simulink model "VehicleModel"  (R2022a)
settings: Solver=VariableStepAuto  StartTime=0.0  StopTime=30  RelTol=1e-3
libraries: simulink x2
settings Model: Creator=raghe  LastModifiedBy=raghe

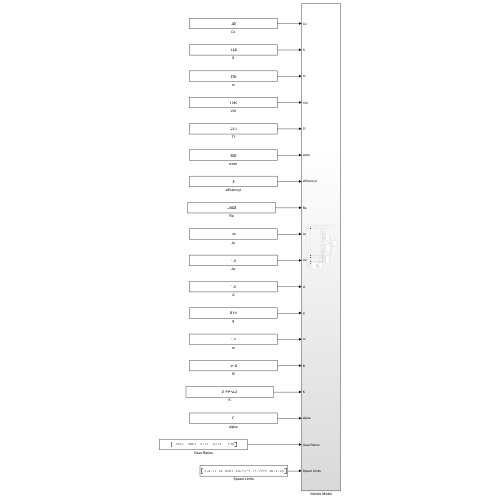
[thumbnail: Simulink's stored preview of the top-level diagram]
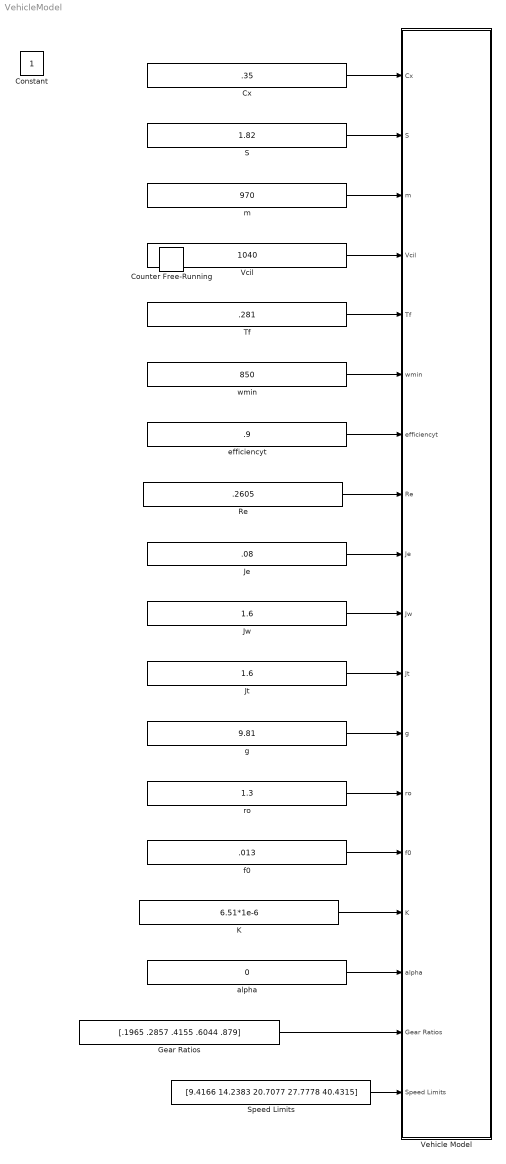
== system VehicleModel ==
  Cx : Constant  Value=.35
  Gear Ratios : Constant  Value=[.1965 .2857 .4155 .6044 .879]
  Je : Constant  Value=.08
  Jt : Constant  Value=1.6
  Jw : Constant  Value=1.6
  K : Constant  Value=6.51*1e-6
  Re : Constant  Value=.2605
  S : Constant  Value=1.82
  Speed Limits : Constant  Value=[9.4166 14.2383 20.7077 27.7778 40.4315]
  Tf : Constant  Value=.281
  Vcil : Constant  Value=1040
  Vehicle Model : Subsystem
  alpha : Constant  Value=0
  efficiencyt : Constant  Value=.9
  f0 : Constant  Value=.013
  g : Constant  Value=9.81
  m : Constant  Value=970
  ro : Constant  Value=1.3
  wmin : Constant  Value=850
  Constant : Constant  IOType=siggen
  Counter Free-Running : simulink/Sources/Counter Free-Running  IOType=siggen  NumBits=16  tsamp=-1
  wires:
  f0/1 -> Vehicle Model/14(f0)
  Vcil/1 -> Vehicle Model/4(Vcil)
  S/1 -> Vehicle Model/2(S)
  g/1 -> Vehicle Model/12(g)
  Re/1 -> Vehicle Model/8(Re)
  Jw/1 -> Vehicle Model/10(Jw)
  efficiencyt/1 -> Vehicle Model/7(efficiencyt)
  Speed Limits/1 -> Vehicle Model/18(Speed Limits)
  Gear Ratios/1 -> Vehicle Model/17(Gear Ratios)
  Je/1 -> Vehicle Model/9(Je)
  Jt/1 -> Vehicle Model/11(Jt)
  Cx/1 -> Vehicle Model/1(Cx)
  ro/1 -> Vehicle Model/13(ro)
  m/1 -> Vehicle Model/3(m)
  K/1 -> Vehicle Model/15(K)
  Tf/1 -> Vehicle Model/5(Tf)
  wmin/1 -> Vehicle Model/6(wmin)
  alpha/1 -> Vehicle Model/16(alpha)

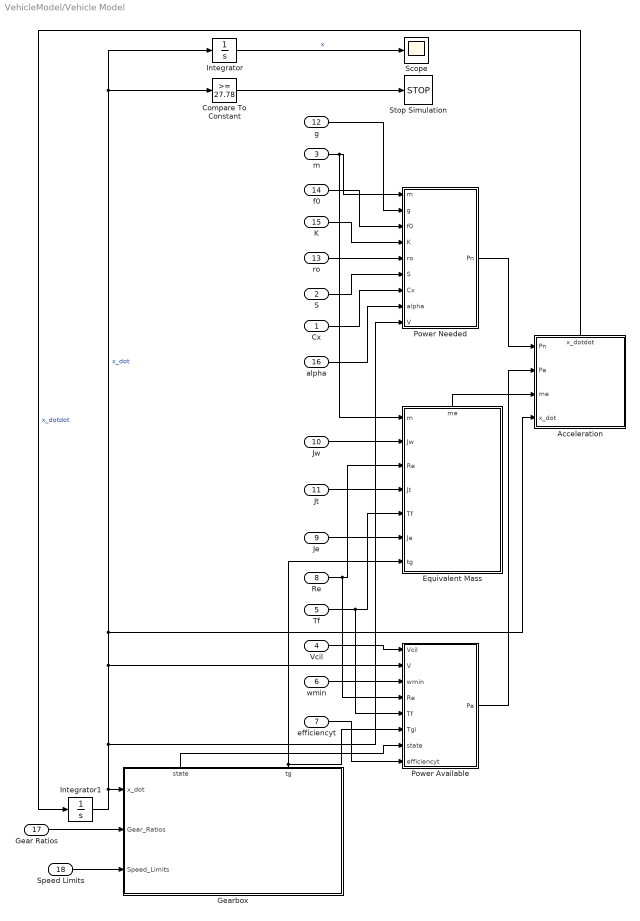
== system VehicleModel/Vehicle Model ==
  Cx : Inport
  S : Inport  Port=2
  m : Inport  Port=3
  Vcil : Inport  Port=4
  Tf : Inport  Port=5
  wmin : Inport  Port=6
  efficiencyt : Inport  Port=7
  Re : Inport  Port=8
  Je : Inport  Port=9
  Jw : Inport  Port=10
  Jt : Inport  Port=11
  g : Inport  Port=12
  ro : Inport  Port=13
  f0 : Inport  Port=14
  K : Inport  Port=15
  alpha : Inport  Port=16
  Gear Ratios : Inport  Port=17
  Speed Limits : Inport  Port=18
  Acceleration : Subsystem
      settings: PortSchema="{\"entries\":[{\"content\":{\"sides\":[{\"content\":{\"connectorIds\":[\"In1\",\"In2\",\"In3\",\"In4\"]},\"type\":\"ConnectorPlacement.EquallySpacedRectSide\",\"uuid\":\"0dac4d62-4e6e-48b9-89ab-502b66d42413\"},{\"content\":{\"connectorIds\":[],\"side\":\"RIGHT\"},\"type\":\"ConnectorPlacement.EquallySpacedRectSide\",\"uuid\":\"bb08bafa-9960-47e7-83c1-b5fcb0a564c6\"},{\"content\":{\"connectorIds\":[\"Out1\"],\"side\":\"TOP\"},\"type\":\"ConnectorPlacement.EquallySpacedRectSide\",\"uuid\":\"4c185d07-b6f8-491a-a2fd-e996dab8f11e\"}]},\"type\":\"ConnectorPlacement.EquallySpacedConnector\",\"uuid\":\"e46381f1-f24e-482b-af6c-f43e86b41e95\"}],\"packageUris\":[\"http://schema.mathworks.com/mf0/Connector/R2020b\"],\"version\":\"1.0\"}"
  Compare To Constant : simulink/Logic and Bit Operations/Compare To Constant  relop=>=  const=27.78  OutDataTypeStr=boolean
  Equivalent Mass : Subsystem
      settings: PortSchema="{\"entries\":[{\"content\":{\"sides\":[{\"content\":{\"connectorIds\":[\"In1\",\"In2\",\"In3\",\"In4\",\"In5\",\"In6\",\"In7\"]},\"type\":\"ConnectorPlacement.EquallySpacedRectSide\",\"uuid\":\"afdafb77-b6a4-4e1f-90ff-c5f4f1bf2fe0\"},{\"content\":{\"connectorIds\":[],\"side\":\"RIGHT\"},\"type\":\"ConnectorPlacement.EquallySpacedRectSide\",\"uuid\":\"5fc42340-ce7c-45bd-a822-e10069a1a8a1\"},{\"content\":{\"connectorIds\":[\"Out1\"],\"side\":\"TOP\"},\"type\":\"ConnectorPlacement.EquallySpacedRectSide\",\"uuid\":\"3dabd7ae-5836-444f-ba7f-aa28a5c4c2aa\"}]},\"type\":\"ConnectorPlacement.EquallySpacedConnector\",\"uuid\":\"25790886-3118-4358-89e2-ebbe2ff8cd9d\"}],\"packageUris\":[\"http://schema.mathworks.com/mf0/Connector/R2020b\"],\"version\":\"1.0\"}"
  Gearbox : Stateflow chart  TreatAsAtomicUnit=on
      settings: PortSchema="{\"entries\":[{\"content\":{\"sides\":[{\"content\":{\"connectorIds\":[\"In1\",\"In2\",\"In3\"]},\"type\":\"ConnectorPlacement.EquallySpacedRectSide\",\"uuid\":\"7b42100c-494e-4f6b-af0e-d741c5c5ef81\"},{\"content\":{\"connectorIds\":[],\"side\":\"RIGHT\"},\"type\":\"ConnectorPlacement.EquallySpacedRectSide\",\"uuid\":\"210b2516-13c7-4261-98c6-692dfef7a0f0\"},{\"content\":{\"connectorIds\":[\"Out2\",\"Out1\"],\"side\":\"TOP\"},\"type\":\"ConnectorPlacement.EquallySpacedRectSide\",\"uuid\":\"dd213d26-eaf8-4fc2-a774-2e7748bf3687\"}]},\"type\":\"ConnectorPlacement.EquallySpacedConnector\",\"uuid\":\"b4102de8-c7c9-4e2e-86dc-7746404cc730\"}],\"packageUris\":[\"http://schema.mathworks.com/mf0/Connector/R2020b\"],\"version\":\"1.0\"}"
  Integrator : Integrator
  Integrator1 : Integrator  InitialCondition=0.1
  Power Available : Subsystem
  Power Needed : Subsystem
  Scope : Scope
  Stop Simulation : Stop
  wires:
  Equivalent Mass/1(me) -> Acceleration/3(me)
  efficiencyt/1 -> Power Available/8(efficiencyt)
  Integrator/1 -> Scope/1  "x"
  Gearbox/2(state) -> Power Available/7(state)
  wmin/1 -> Power Available/3(wmin)
  Power Available/1(Pa) -> Acceleration/2(Pa)
  Compare To Constant/1 -> Stop Simulation/1
  S/1 -> Power Needed/6(S)
  Vcil/1 -> Power Available/1(Vcil)
  Power Needed/1(Pn) -> Acceleration/1(Pn)
  Je/1 -> Equivalent Mass/6(Je)
  Jt/1 -> Equivalent Mass/4(Jt)
  Gearbox/1(tg) -> Equivalent Mass/7(tg), Power Available/6(Tgi)
  Jw/1 -> Equivalent Mass/2(Jw)
  alpha/1 -> Power Needed/8(alpha)
  Cx/1 -> Power Needed/7(Cx)
  ro/1 -> Power Needed/5(ro)
  K/1 -> Power Needed/4(K)
  f0/1 -> Power Needed/3(f0)
  g/1 -> Power Needed/2(g)
  Acceleration/1(x_dotdot) -> Integrator1/1  "x_dotdot"
  m/1 -> Power Needed/1(m), Equivalent Mass/1(m)
  Tf/1 -> Power Available/5(Tf), Equivalent Mass/5(Tf)
  Re/1 -> Power Available/4(Re), Equivalent Mass/3(Re)
  Integrator1/1 -> Compare To Constant/1, Integrator/1, Acceleration/4(x_dot), Power Available/2(V), Power Needed/9(V), Gearbox/1(x_dot)  "x_dot"
  Gear Ratios/1 -> Gearbox/2(Gear_Ratios)
  Speed Limits/1 -> Gearbox/3(Speed_Limits)

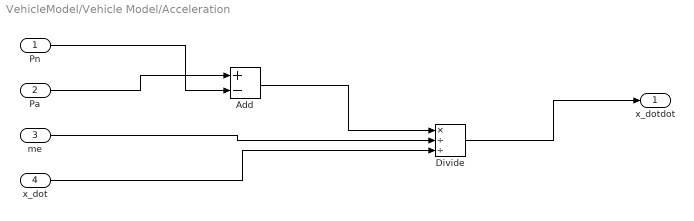
== system VehicleModel/Vehicle Model/Acceleration ==
  Pn : Inport
  Pa : Inport  Port=2
  me : Inport  Port=3
  x_dot : Inport  Port=4
  Add : Sum  Inputs=+-
  Divide : Product  Inputs=*//
  x_dotdot : Outport
  wires:
  Pa/1 -> Add/1
  Pn/1 -> Add/2
  x_dot/1 -> Divide/3
  me/1 -> Divide/2
  Add/1 -> Divide/1
  Divide/1 -> x_dotdot/1

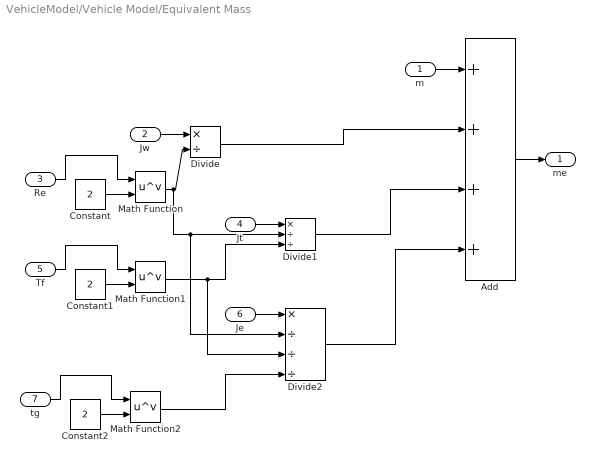
== system VehicleModel/Vehicle Model/Equivalent Mass ==
  m : Inport
  Jw : Inport  Port=2
  Re : Inport  Port=3
  Jt : Inport  Port=4
  Tf : Inport  Port=5
  Je : Inport  Port=6
  tg : Inport  Port=7
  Add : Sum  Inputs=++++
  Constant : Constant  Value=2
  Constant1 : Constant  Value=2
  Constant2 : Constant  Value=2
  Divide : Product  Inputs=*/
  Divide1 : Product  Inputs=*//
  Divide2 : Product  Inputs=*///
  Math Function : Math  Operator=pow
  Math Function1 : Math  Operator=pow
  Math Function2 : Math  Operator=pow
  me : Outport
  wires:
  Re/1 -> Math Function/1
  Constant/1 -> Math Function/2
  Jw/1 -> Divide/1
  Math Function/1 -> Divide2/2, Divide1/2, Divide/2
  Jt/1 -> Divide1/1
  Constant1/1 -> Math Function1/2
  Tf/1 -> Math Function1/1
  Math Function1/1 -> Divide2/3, Divide1/3
  Math Function2/1 -> Divide2/4
  Constant2/1 -> Math Function2/2
  Je/1 -> Divide2/1
  tg/1 -> Math Function2/1
  m/1 -> Add/1
  Divide/1 -> Add/2
  Divide1/1 -> Add/3
  Divide2/1 -> Add/4
  Add/1 -> me/1

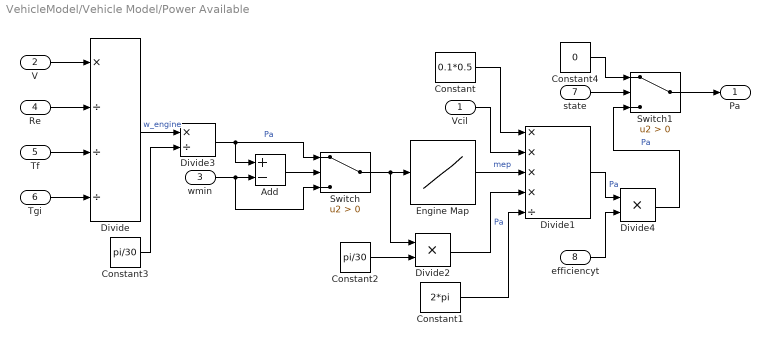
== system VehicleModel/Vehicle Model/Power Available ==
  Vcil : Inport
  V : Inport  Port=2
  wmin : Inport  Port=3
  Re : Inport  Port=4
  Tf : Inport  Port=5
  Tgi : Inport  Port=6
  state : Inport  Port=7
  efficiencyt : Inport  Port=8
  Add : Sum  Inputs=+-
  Constant : Constant  Value=0.1*0.5
  Constant1 : Constant  Value=2*pi
  Constant2 : Constant  Value=pi/30
  Constant3 : Constant  Value=pi/30
  Constant4 : Constant  Value=0
  Divide : Product  Inputs=*///
  Divide1 : Product  Inputs=****/
  Divide2 : Product  Inputs=**
  Divide3 : Product  Inputs=*/
  Divide4 : Product  Inputs=**
  Engine Map : Lookup_n-D  NumberOfTableDimensions=1  BreakpointsForDimension1=[1000;1500;2000;2500;3000;3250;3500;4000;4500;5000;5500;6000;6500]  Table=[5.99;8.58;8.84;9.33;9.51;9.67;9.61;9.63;9.48;8.93;8.25;7.79;7.12]  InternalRulePriority=Speed  RndMeth=Simplest
  Switch : Switch  Criteria=u2 > Threshold  SaturateOnIntegerOverflow=off  InputSameDT=off
  Switch1 : Switch  Criteria=u2 > Threshold  SaturateOnIntegerOverflow=off  InputSameDT=off
  Pa : Outport
  wires:
  Re/1 -> Divide/2
  Switch1/1 -> Pa/1
  Constant3/1 -> Divide3/2
  Divide/1 -> Divide3/1  "w_engine"
  Constant4/1 -> Switch1/1
  Tf/1 -> Divide/3
  state/1 -> Switch1/2
  V/1 -> Divide/1
  Tgi/1 -> Divide/4
  Vcil/1 -> Divide1/2
  Constant1/1 -> Divide1/5
  wmin/1 -> Switch/3, Add/2
  Add/1 -> Switch/2
  Constant2/1 -> Divide2/2
  Constant/1 -> Divide1/1
  Divide2/1 -> Divide1/4  "Pa"
  Engine Map/1 -> Divide1/3  "mep"
  Divide3/1 -> Add/1, Switch/1  "Pa"
  Switch/1 -> Divide2/1, Engine Map/1
  Divide1/1 -> Divide4/1  "Pa"
  efficiencyt/1 -> Divide4/2
  Divide4/1 -> Switch1/3  "Pa"

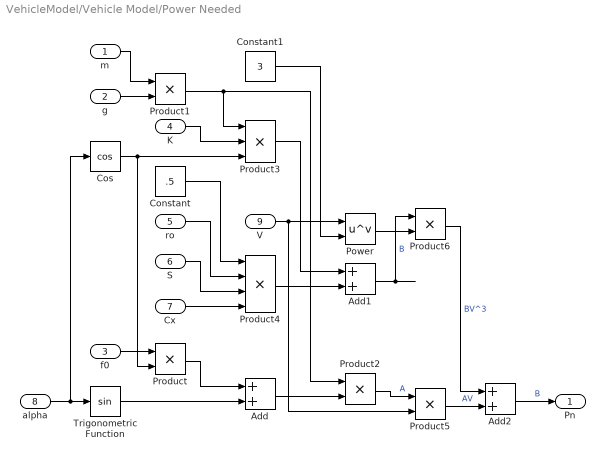
== system VehicleModel/Vehicle Model/Power Needed ==
  m : Inport
  g : Inport  Port=2
  f0 : Inport  Port=3
  K : Inport  Port=4
  ro : Inport  Port=5
  S : Inport  Port=6
  Cx : Inport  Port=7
  alpha : Inport  Port=8
  V : Inport  Port=9
  Add : Sum
  Add1 : Sum
  Add2 : Sum
  Constant : Constant  Value=.5
  Constant1 : Constant  Value=3
  Cos : Trigonometry  Operator=cos
  Power : Math  Operator=pow
  Product{,1..2,5..6} (5 alike) : Product
  Product3 : Product  Inputs=3
  Product4 : Product  Inputs=4
  Trigonometric Function : Trigonometry
  Pn : Outport
  wires:
  Add2/1 -> Pn/1  "B"
  Product3/1 -> Add1/1
  S/1 -> Product4/3
  Product6/1 -> Add2/1  "BV^3"
  Power/1 -> Product6/2
  Constant1/1 -> Power/2
  Product5/1 -> Add2/2  "AV"
  Product4/1 -> Add1/2
  Cx/1 -> Product4/4
  ro/1 -> Product4/2
  alpha/1 -> Cos/1, Trigonometric Function/1
  Constant/1 -> Product4/1
  K/1 -> Product3/2
  Product2/1 -> Product5/1  "A"
  Add/1 -> Product2/2
  g/1 -> Product1/2
  m/1 -> Product1/1
  Trigonometric Function/1 -> Add/2
  Product/1 -> Add/1
  f0/1 -> Product/1
  V/1 -> Product5/2, Power/1
  Add1/1 -> Product6/1  "B"
  Product1/1 -> Product2/1, Product3/1
  Cos/1 -> Product/2, Product3/3

== stateflow chart VehicleModel/Vehicle Model/Gearbox ==
  state gear_state [parallel]
    entry:
    i = 1;
    settings: executionOrder=1
    state engage
      tg = Gear_Ratios(i);
      up_th = Speed_Limits(i);
      if(i == 1)
      down_th = 0;
      else
      down_th = Speed_Limits(i-1);
      end
    engage -> engage [order 1] : UP{i = i + 1;}
    engage -> engage [order 2] : DOWN{i = i - 1;}
  state selection_state [parallel]
    settings: executionOrder=2
    state steady
      entry:
      state = 0;
    state downshifting
      entry:
      state = 1;
    state upshifting
      entry:
      state = 1;
    (default) -> steady
    steady -> downshifting [order 2] : [x_dot < down_th]
    steady -> upshifting [order 1] : [x_dot > up_th]
    downshifting -> steady : after(1, sec){send(DOWN, gear_state)}
    upshifting -> steady : after(1, sec){send(UP, gear_state)}
  data: x_dot input; tg output; state output; down_th local double size=1; up_th local double size=1; Gear_Ratios input; Speed_Limits input; i local
  events: UP local FUNCTION_CALL_EVENT; DOWN local FUNCTION_CALL_EVENT
